simulink library "vhcl4turbAndrewMess_cl"  (R2022a)
settings: Solver=VariableStepAuto  StartTime=0.0  StopTime=10.0  RelTol=1e-3
undefined symbols (not defined in the file): env, thrSwitch, VEHICLE, vhcl, XiTotA, XiTotD
libraries: vrlib x4, addedMass_cl x1, pathFollowingCtrlAoATurbDiscrete_cl x1, dynamicPressure_ul x1, courseFollowLookAhead_cl x1, sharedutil x1, gnd2TanRotation_ul x1, pathGeometry_ul x1, velocityAngle_ul x1, alphaBeta_ul x1, dragTurbine x1, Copy_of_fluidDynamicSurface_cl x1
settings Model: Creator=mcobb  LastModifiedBy=adabney
settings SolverCC: AlgebraicLoopSolver=TrustRegion
settings DataIOCC: ReturnWorkspaceOutputs=off
settings DebuggingCC: UnconnectedInputMsg=warning  UnconnectedOutputMsg=warning  UnconnectedLineMsg=warning  SFMachineParentedDataDiag=warning  ArithmeticOperatorsInVariantConditions=warning
settings SFSimCC: CustomCodeUndefinedFunction=UseInterfaceOnly

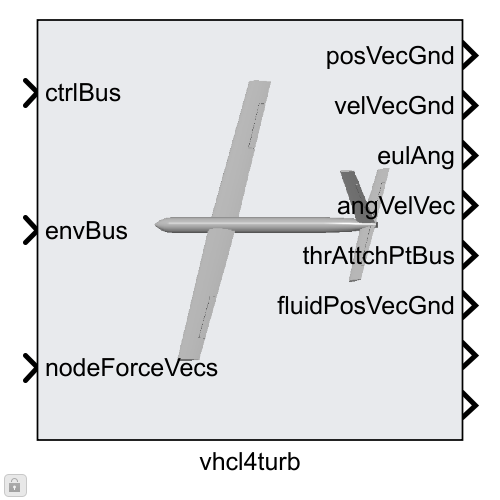
[thumbnail: Simulink's stored preview of the top-level diagram]
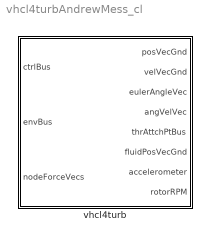
== system vhcl4turbAndrewMess_cl ==
  vhcl4turb : Subsystem  VariantControl=strcmpi(VEHICLE,'vehicleManta')  mask{vcl=vhcl, rho=env.water.density.Value, grav=env.gravAccel.Value}
      mask prompts: vcl "Vehicle"; rho "Density"; grav "Gravity"
      mask init:
      | numTurb = vcl.numTurbines.Value;
      | 
      | if numTurb == 0
      |     turbInd = [];
      |     gradInd = [6:11];
      | else
      |     turbInd = [1:numTurb]+5;
      |     gradInd = [6:11]+numTurb;
      | end
      | 
      | flowPoll = ones(1,numTurb+11);
      mask DialogControl Container9 Prompt: General
      mask DialogControl Container5 Prompt: Vehicle object (OCT.vehicle)
      mask DialogControl ParameterGroupVar Prompt: Environment Object (OCT.env)
      mask Display:
      | image('kite2.PNG',[0 0 700 700]/4,'on')
      | 
      | port_label('input',1,'ctrlBus')
      | port_label('input',2,'envBus')
      | port_label('input',3,'nodeForceVecs')
      | 
      | port_label('output',1,'posVecGnd')
      | port_label('output',2,'velVecGnd')
      | port_label('output',3,'eulAng')
      | port_label('output',4,'angVelVec')
      | port_label('output',5,'thrAttchPtBus')
      | port_label('output',6,'fluidPosVecGnd')

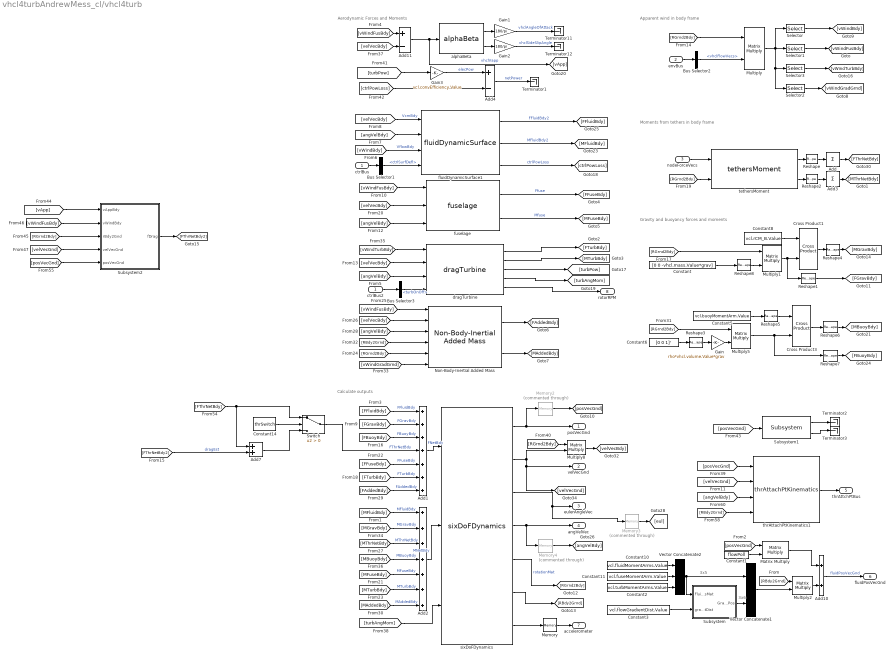
== system vhcl4turbAndrewMess_cl/vhcl4turb ==
  note: 3x6
  note: 3x5
  note: Calculate outputs
  note: Apparent wind in body frame
  note: Gravity and buoyancy forces and moments
  note: Moments from tethers in body frame
  note: Aerodynamic Forces and Moments
  ctrlBus : Inport  OutDataTypeStr=Bus: fltCtrlBus
  envBus : Inport  Port=2  OutDataTypeStr=Bus: envBus
  nodeForceVecs : Inport  Port=3
  Add : Sum  Inputs=+  CollapseMode=Specified dimension  CollapseDim=2
  Add1 : Sum  Inputs=+++++++
  Add10 : Sum
  Add11 : Sum  Inputs=+-
  Add2 : Sum  Inputs=+++++++
  Add3 : Sum  Inputs=+  CollapseMode=Specified dimension  CollapseDim=2
  Add4 : Sum  Inputs=+-
  Add7 : Sum
  Bus Selector1 : BusSelector  OutputSignals=ctrlSurfDefl
  Bus Selector2 : BusSelector  OutputSignals=vhclFlowVecs
  Bus Selector3 : BusSelector  OutputSignals=turbOnOff
  Constant : Constant  Value=[0 0 -vhcl.mass.Value*grav]
  Constant1 : Constant  Value=flowPoll  VectorParams1D=off
  Constant10 : Constant  Value=vcl.fluidMomentArms.Value
  Constant11 : Constant  Value=vcl.fuseMomentArm.Value
  Constant14 : Constant  Value=thrSwitch
  Constant2 : Constant  Value=vcl.turbMomentArms.Value
  Constant3 : Constant  Value=vcl.flowGradientDist.Value
  Constant5 : Constant  Value=vcl.buoyMomentArm.Value
  Constant6 : Constant  Value=[0 0 1]'
  Constant8 : Constant  Value=vcl.rCM_B.Value
  Cross Product1 : vrlib/Utilities/Cross Product
  Cross Product3 : vrlib/Utilities/Cross Product
  Gain : Gain  Gain=rho*vhcl.volume.Value*grav
  Gain1 : Gain  Gain=180/pi
  Gain2 : Gain  Gain=180/pi
  Gain3 : Gain  Gain=vcl.convEfficiency.Value
  Matrix Multiply : Product  Multiplication=Matrix(*)
  Memory : Memory
  Memory2 : Memory  Commented=through  InitialCondition=vcl.initPosVecGnd.Value
  Memory3 : Memory  Commented=through  InitialCondition=vcl.initEulAng.Value
  Memory4 : Memory  Commented=through  InitialCondition=vcl.initAngVelVec.Value
  Multiply{,1..2,5,8} (5 alike) : Product  Multiplication=Matrix(*)
  Non-Body-Inertial Added Mass : addedMass_cl/Non-Body-Inertial Added Mass  MaMat=vcl.Ma6x6_LE.Value  rB_LE=vcl.rB_LE.Value  gradDist=vcl.flowGradientDist.Value
  Reshape : Reshape  OutputDimensionality=Customize  OutputDimensions=[3 vcl.numTethers.Value]
  Reshape{1,3..8} (7 alike) : Reshape  OutputDimensionality=Column vector (2-D)
  Reshape2 : Reshape  OutputDimensionality=Customize  OutputDimensions=[3 vcl.numTethers.Value]
  Selector : Selector  NumberOfDimensions=2  InputPortWidth=3  IndexOptions=Select all,Index vector (dialog)  Indices=[1 3],1:4  OutputSizes=1,1
  Selector1 : Selector  NumberOfDimensions=2  InputPortWidth=3  IndexOptions=Select all,Index vector (dialog)  Indices=[1 3],5  OutputSizes=1,1
  Selector2 : Selector  NumberOfDimensions=2  InputPortWidth=3  IndexOptions=Select all,Index vector (dialog)  Indices=[1 3],gradInd  OutputSizes=1,1
  Selector3 : Selector  NumberOfDimensions=2  InputPortWidth=3  IndexOptions=Select all,Index vector (dialog)  Indices=[1 3],turbInd  OutputSizes=1,1
  Subsystem : Subsystem
  Subsystem1 : pathFollowingCtrlAoATurbDiscrete_cl/pathFollowingCtrlAoATurbDiscrete/Subsystem  SystemSampleTime=-1  VariantActivationTime=update diagram  Latency=0  AutoFrameSizeCalculation=off
  Subsystem2 : Subsystem  mask{vcl=vcl}
      mask prompts: vcl "Vehicle"
  Switch : Switch  Criteria=u2 > Threshold  SaturateOnIntegerOverflow=off  InputSameDT=off
  Terminator{1..3,11..12} (5 alike) : Terminator
  Vector Concatenate1 : Concatenate  Mode=Multidimensional array  ConcatenateDimension=2
  Vector Concatenate2 : Concatenate  NumInputs=3  Mode=Multidimensional array  ConcatenateDimension=2
  alphaBeta : alphaBeta_ul/alphaBeta  SystemSampleTime=-1  VariantActivationTime=update diagram  Latency=0  AutoFrameSizeCalculation=off
  ctrlBus2 : InportShadow  OutDataTypeStr=Bus: fltCtrlBus
  dragTurbine : dragTurbine/dragTurbine  vhcl=vcl  thr=0
  fluidDynamicSurface1 : Copy_of_fluidDynamicSurface_cl/fluidDynamicSurface  vcl=vcl  fluidDensity=env.water.density.Value  fluidMomentArms=vcl.fluidMomentArms.Value  fluidRefArea=vcl.fluidRefArea.Value  wingTips=vcl.wingTipPositions.Value
  fuselage : fuselage_cl/fuselage  momArm=vcl.fuseMomentArm.Value  fus=vcl.fuse  fusRhoDa=rho
  sixDoFDynamics : sixDoFDynamics_cl/sixDoFDynamics  vcl=vcl
  tethersMoment : tethersMoment_cl/tethersMoment  arms=vcl.struct('OCT.thrAttch')
  thrAttachPtKinematics1 : thrAttachPtKinematics_ul/thrAttachPtKinematics  atchPts=vcl.struct('OCT.thrAttch')
  posVecGnd : Outport  VectorParamsAs1DForOutWhenUnconnected=off
  velVecGnd : Outport  Port=2  VectorParamsAs1DForOutWhenUnconnected=off
  eulerAngleVec : Outport  Port=3  VectorParamsAs1DForOutWhenUnconnected=off
  angVelVec : Outport  Port=4  VectorParamsAs1DForOutWhenUnconnected=off
  thrAttchPtBus : Outport  Port=5  VectorParamsAs1DForOutWhenUnconnected=off
  fluidPosVecGnd : Outport  Port=6  VectorParamsAs1DForOutWhenUnconnected=off
  accelerometer : Outport  Port=7
  rotorRPM : Outport  Port=8
  wires:
  sixDoFDynamics/3 -> Memory3/1, eulerAngleVec/1
  sixDoFDynamics/1 -> Memory2/1, posVecGnd/1
  sixDoFDynamics/2 -> [velVecGnd], velVecGnd/1, Multiply8/2
  thrAttachPtKinematics1/1 -> thrAttchPtBus/1
  [vWindFusBdy] -> fuselage/1
  [velVecBdy] -> fuselage/2
  [angVelBdy] -> fuselage/3
  [vWindTurbBdy] -> dragTurbine/1
  [velVecBdy] -> dragTurbine/2
  [angVelBdy] -> dragTurbine/3
  [vWindFusBdy] -> Non-Body-Inertial Added Mass/1
  [velVecBdy] -> Non-Body-Inertial Added Mass/2
  [angVelBdy] -> Non-Body-Inertial Added Mass/3
  [RBdy2Grnd] -> Non-Body-Inertial Added Mass/4
  [RGrnd2Bdy] -> Non-Body-Inertial Added Mass/5
  [vWindGradGrnd] -> Non-Body-Inertial Added Mass/6
  Constant6/1 -> Reshape3/1
  Reshape3/1 -> Gain/1
  [RGrnd2Bdy] -> Multiply5/1
  Gain/1 -> Multiply5/2
  Constant5/1 -> Reshape5/1
  Reshape5/1 -> Cross Product3/1
  Cross Product3/1 -> Reshape6/1
  Reshape6/1 -> [MBuoyBdy]
  Multiply5/1 -> Reshape7/1, Cross Product3/2
  Reshape7/1 -> [FBuoyBdy]
  Reshape1/1 -> [FGravBdy]
  Multiply1/1 -> Reshape1/1, Cross Product1/2
  fuselage/1 -> [FFuseBdy]  "Ffuse"
  fuselage/2 -> [MFuseBdy]  "Mfuse"
  Constant/1 -> Reshape8/1
  [RGrnd2Bdy] -> Multiply1/1
  Reshape8/1 -> Multiply1/2
  Constant8/1 -> Cross Product1/1
  Cross Product1/1 -> Reshape4/1
  Reshape4/1 -> [MGravBdy]
  [RGrnd2Bdy] -> tethersMoment/2
  nodeForceVecs/1 -> tethersMoment/1
  tethersMoment/1 -> Reshape/1
  tethersMoment/2 -> Reshape2/1
  Reshape/1 -> Add/1
  Reshape2/1 -> Add3/1
  Add/1 -> [FThrNetBdy]
  Add3/1 -> [MThrNetBdy]
  [RGrnd2Bdy] -> Multiply/1
  envBus/1 -> Bus Selector2/1
  Bus Selector2/1 -> Multiply/2  "<vhclFlowVecs>"
  Multiply/1 -> Selector/1, Selector2/1, Selector3/1, Selector1/1
  Selector/1 -> [vWindBdy]
  Selector1/1 -> [vWindFusBdy]
  Selector2/1 -> [vWindGradGrnd]
  [RGrnd2Bdy] -> Multiply8/1
  Multiply8/1 -> [velVecBdy]
  [FFluidBdy] -> Add1/1  "FFluidBdy"
  [FGravBdy] -> Add1/2  "FGravBdy"
  [FBuoyBdy] -> Add1/3  "FBuoyBdy"
  Switch/1 -> Add1/4  "FThrNetBdy"
  [FFuseBdy] -> Add1/5  "FFuseBdy"
  [FTurbBdy] -> Add1/6  "FTurbBdy"
  [FAddedBdy] -> Add1/7  "FAddedBdy"
  Add1/1 -> sixDoFDynamics/1  "FNetBdy"
  [MFluidBdy] -> Add2/1  "MFluidBdy"
  [MGravBdy] -> Add2/2  "MGravBdy"
  [MThrNetBdy] -> Add2/3  "MThrNetBdy"
  [MBuoyBdy] -> Add2/4  "MBuoyBdy"
  [MFuseBdy] -> Add2/5  "MFuseBdy"
  [MTurbBdy] -> Add2/6  "MTurbBdy"
  [MAddedBdy] -> Add2/7  "MAddedBdy"
  Add2/1 -> sixDoFDynamics/2  "MNetBdy"
  sixDoFDynamics/5 -> [RGrnd2Bdy]  "rotationMat"
  sixDoFDynamics/6 -> [RBdy2Grnd]
  [posVecGnd] -> thrAttachPtKinematics1/1
  [velVecGnd] -> thrAttachPtKinematics1/2
  [angVelBdy] -> thrAttachPtKinematics1/3
  [RBdy2Grnd] -> thrAttachPtKinematics1/4
  Constant10/1 -> Vector Concatenate2/1
  Constant11/1 -> Vector Concatenate2/2
  Vector Concatenate2/1 -> Vector Concatenate1/1, Subsystem/1(FluidCentPosMat)
  Constant3/1 -> Subsystem/2(gradientDist)
  Subsystem/1(GradientFlowPos) -> Vector Concatenate1/2
  sixDoFDynamics/4 -> Memory4/1, angVelVec/1
  Vector Concatenate1/1 -> Multiply2/2
  [RBdy2Grnd] -> Multiply2/1
  Multiply2/1 -> Add10/2
  Matrix Multiply/1 -> Add10/1
  Add10/1 -> fluidPosVecGnd/1  "fluidPosVecGnd"
  Constant1/1 -> Matrix Multiply/2
  [posVecGnd] -> Matrix Multiply/1
  Bus Selector3/1 -> dragTurbine/4  "<turbOnOff>"
  ctrlBus2/1 -> Bus Selector3/1
  Constant2/1 -> Vector Concatenate2/3
  Selector3/1 -> [vWindTurbBdy]
  dragTurbine/1 -> [FTurbBdy]
  dragTurbine/2 -> [MTurbBdy]
  dragTurbine/3 -> [turbPow]
  dragTurbine/4 -> [turbAngMom]
  dragTurbine/5 -> rotorRPM/1
  fluidDynamicSurface1/1 -> [FFluidBdy]  "FFluidBdy2"
  Gain3/1 -> Add4/1  "elecPow"
  [ctrlPowLoss] -> Add4/2
  [turbPow] -> Gain3/1
  fluidDynamicSurface1/3 -> [ctrlPowLoss]  "ctrlPowLoss"
  [angVelBdy] -> fluidDynamicSurface1/2
  [vWindBdy] -> fluidDynamicSurface1/3  "VflowBdy"
  [velVecBdy] -> fluidDynamicSurface1/1  "VcmBdy"
  fluidDynamicSurface1/2 -> [MFluidBdy]  "MFluidBdy2"
  Bus Selector1/1 -> fluidDynamicSurface1/4  "<ctrlSurfDefl>"
  Gain2/1 -> Terminator12/1  "vhclSideSlipAngle"
  alphaBeta/1 -> Gain1/1
  Add4/1 -> Terminator1/1  "netPower"
  Gain1/1 -> Terminator11/1  "vhclAngleOfAttack"
  [vWindFusBdy] -> Add11/1
  Add11/1 -> [vApp], alphaBeta/1  "vhclVapp"
  alphaBeta/2 -> Gain2/1
  ctrlBus/1 -> Bus Selector1/1
  Memory/1 -> accelerometer/1
  sixDoFDynamics/7 -> Memory/1
  [turbAngMom] -> sixDoFDynamics/3
  [posVecGnd] -> Subsystem1/1
  Subsystem1/1 -> Terminator2/1
  Subsystem1/2 -> Terminator3/1
  Non-Body-Inertial Added Mass/1 -> [FAddedBdy]
  Non-Body-Inertial Added Mass/2 -> [MAddedBdy]
  [velVecBdy] -> Add11/2
  Memory2/1 -> [posVecGnd]
  Memory3/1 -> [eul]
  Memory4/1 -> [angVelBdy]
  [FThrNetBdy2] -> Add7/2  "dragEst"
  Constant14/1 -> Switch/2
  [FThrNetBdy] -> Add7/1, Switch/1
  Add7/1 -> Switch/3
  [vApp] -> Subsystem2/1(vAppBdy)
  [vWindFusBdy] -> Subsystem2/2(vWindBdy)
  [velVecGnd] -> Subsystem2/4(velVecGnd)
  [posVecGnd] -> Subsystem2/5(posVecGnd)
  [RGrnd2Bdy] -> Subsystem2/3(rBdy2Gnd)
  Subsystem2/1(fDrag) -> [FThrNetBdy2]

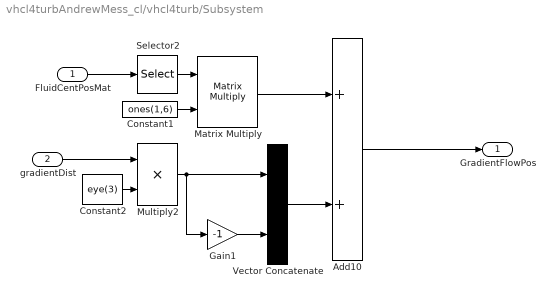
== system vhcl4turbAndrewMess_cl/vhcl4turb/Subsystem ==
  FluidCentPosMat : Inport
  gradientDist : Inport  Port=2
  Add10 : Sum
  Constant1 : Constant  Value=ones(1,6)  VectorParams1D=off
  Constant2 : Constant  Value=eye(3)
  Gain1 : Gain  Gain=-1
  Matrix Multiply : Product  Multiplication=Matrix(*)
  Multiply2 : Product
  Selector2 : Selector  NumberOfDimensions=2  InputPortWidth=3  IndexOptions=Select all,Index vector (dialog)  Indices=[1 3],5  OutputSizes=1,1
  Vector Concatenate : Concatenate  Mode=Multidimensional array  ConcatenateDimension=2
  GradientFlowPos : Outport  VectorParamsAs1DForOutWhenUnconnected=off
  wires:
  FluidCentPosMat/1 -> Selector2/1
  Vector Concatenate/1 -> Add10/2
  Selector2/1 -> Matrix Multiply/1
  Multiply2/1 -> Gain1/1, Vector Concatenate/1
  Constant1/1 -> Matrix Multiply/2
  Matrix Multiply/1 -> Add10/1
  Gain1/1 -> Vector Concatenate/2
  Constant2/1 -> Multiply2/2
  Add10/1 -> GradientFlowPos/1
  gradientDist/1 -> Multiply2/1

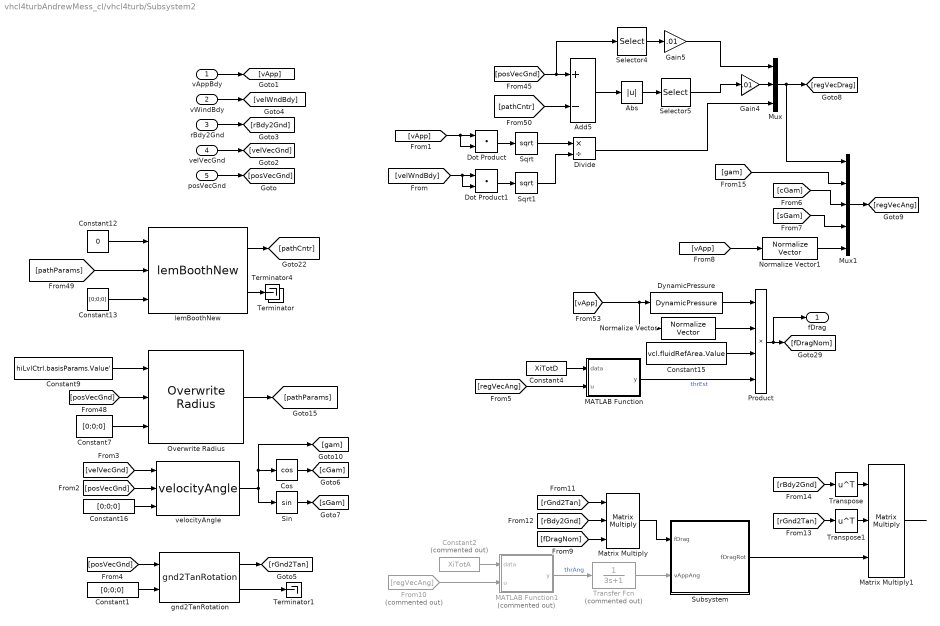
== system vhcl4turbAndrewMess_cl/vhcl4turb/Subsystem2 ==
  vAppBdy : Inport
  vWindBdy : Inport  Port=2
  rBdy2Gnd : Inport  Port=3
  velVecGnd : Inport  Port=4
  posVecGnd : Inport  Port=5
  Abs : Abs  SaturateOnIntegerOverflow=off
  Add5 : Sum  Inputs=+-
  Constant{1,7,13,16} (4 alike) : Constant  Value=[0;0;0]  VectorParams1D=off
  Constant12 : Constant  Value=0
  Constant15 : Constant  Value=vcl.fluidRefArea.Value
  Constant2 : Constant  Commented=on  Value=XiTotA
  Constant4 : Constant  Value=XiTotD
  Constant9 : Constant  Value=hiLvlCtrl.basisParams.Value'  VectorParams1D=off
  Cos : Trigonometry  Operator=cos
  Divide : Product  Inputs=*/
  Dot Product : DotProduct  OutDataTypeStr=Inherit: Inherit via internal rule
  Dot Product1 : DotProduct  OutDataTypeStr=Inherit: Inherit via internal rule
  DynamicPressure : dynamicPressure_ul/DynamicPressure  rho=1000
  From10 : From  Commented=on  GotoTag=regVecAng
  Gain4 : Gain  Gain=.01
  Gain5 : Gain  Gain=.01
  MATLAB Function : MATLAB Function  TreatAsAtomicUnit=on
  MATLAB Function1 : MATLAB Function  Commented=on  TreatAsAtomicUnit=on
  Matrix Multiply : Product  Inputs=3  Multiplication=Matrix(*)
  Matrix Multiply1 : Product  Inputs=3  Multiplication=Matrix(*)
  Mux : Mux  Inputs=3
  Mux1 : Mux  Inputs=5
  Normalize Vector : vrlib/Utilities/Normalize Vector  maxzero=0
  Normalize Vector1 : vrlib/Utilities/Normalize Vector  maxzero=0
  Overwrite Radius : courseFollowLookAhead_cl/courseFollowLookAhead/Overwrite Radius  SystemSampleTime=-1  VariantActivationTime=update diagram  Latency=0  AutoFrameSizeCalculation=off
  Product : Product  Inputs=4
  Selector4 : Selector  InputPortWidth=3  IndexOptions=Index vector (dialog)  Indices=3  OutputSizes=1
  Selector5 : Selector  InputPortWidth=3  IndexOptions=Index vector (dialog)  Indices=[2 3]  OutputSizes=1
  Sin : Trigonometry
  Sqrt : Sqrt
  Sqrt1 : Sqrt
  Subsystem : Subsystem
  Terminator : Terminator
  Terminator1 : Terminator
  Terminator4 : Terminator
  Transfer Fcn : TransferFcn  Commented=on  Denominator=[3 1]
  Transpose : Math  Operator=transpose
  Transpose1 : Math  Operator=transpose
  gnd2TanRotation : gnd2TanRotation_ul/gnd2TanRotation  SystemSampleTime=-1  VariantActivationTime=update diagram  Latency=0  AutoFrameSizeCalculation=off
  lemBoothNew : pathGeometry_ul/pathGeometry/lemBoothNew  SystemSampleTime=-1  VariantControl=VSS_pathGeometry_lemBoothNew  VariantActivationTime=update diagram  Latency=0  AutoFrameSizeCalculation=off
  velocityAngle : velocityAngle_ul/velocityAngle  SystemSampleTime=-1  VariantActivationTime=update diagram  Latency=0  AutoFrameSizeCalculation=off
  fDrag : Outport
  wires:
  [posVecGnd] -> Overwrite Radius/2
  lemBoothNew/2 -> Terminator4/1
  Overwrite Radius/1 -> [pathParams]
  Selector4/1 -> Gain5/1
  Abs/1 -> Selector5/1
  Constant12/1 -> lemBoothNew/1
  Gain4/1 -> Mux/2
  Constant13/1 -> lemBoothNew/3
  Add5/1 -> Abs/1
  Dot Product1/1 -> Sqrt1/1
  lemBoothNew/1 -> [pathCntr]
  Gain5/1 -> Mux/1
  Sqrt1/1 -> Divide/2
  Sqrt/1 -> Divide/1
  Dot Product/1 -> Sqrt/1
  velocityAngle/1 -> [gam], Cos/1, Sin/1
  Divide/1 -> Mux/3
  [posVecGnd] -> Selector4/1, Add5/1
  Constant16/1 -> velocityAngle/3
  Constant7/1 -> Overwrite Radius/3
  Constant9/1 -> Overwrite Radius/1
  Mux/1 -> Mux1/1, [regVecDrag]
  [pathCntr] -> Add5/2
  [pathParams] -> lemBoothNew/2
  Selector5/1 -> Gain4/1
  posVecGnd/1 -> [posVecGnd]
  vAppBdy/1 -> [vApp]
  vWindBdy/1 -> [velWndBdy]
  [velWndBdy] -> Dot Product1/2, Dot Product1/1
  [vApp] -> Dot Product/2, Dot Product/1
  rBdy2Gnd/1 -> [rBdy2Gnd]
  velVecGnd/1 -> [velVecGnd]
  [posVecGnd] -> velocityAngle/2
  [velVecGnd] -> velocityAngle/1
  Cos/1 -> [cGam]
  Sin/1 -> [sGam]
  gnd2TanRotation/1 -> [rGnd2Tan]
  [posVecGnd] -> gnd2TanRotation/1
  Constant1/1 -> gnd2TanRotation/2
  gnd2TanRotation/2 -> Terminator1/1
  [vApp] -> Normalize Vector/1, DynamicPressure/1
  Product/1 -> fDrag/1, [fDragNom]
  Normalize Vector/1 -> Product/2
  Constant15/1 -> Product/3
  MATLAB Function/1(y) -> Product/4  "thrEst"
  DynamicPressure/1 -> Product/1
  Constant4/1 -> MATLAB Function/1(data)
  [regVecAng] -> MATLAB Function/2(u)
  [cGam] -> Mux1/3
  [sGam] -> Mux1/4
  [vApp] -> Normalize Vector1/1
  Mux1/1 -> [regVecAng]
  From10/1 -> MATLAB Function1/2(u)
  Constant2/1 -> MATLAB Function1/1(data)
  MATLAB Function1/1(y) -> Transfer Fcn/1  "thrAng"
  Subsystem/1(fDragRot) -> Matrix Multiply1/3
  [fDragNom] -> Matrix Multiply/3
  [rBdy2Gnd] -> Matrix Multiply/2
  [rGnd2Tan] -> Matrix Multiply/1
  Matrix Multiply/1 -> Subsystem/1(fDrag)
  [rBdy2Gnd] -> Transpose/1
  Transpose/1 -> Matrix Multiply1/1
  [rGnd2Tan] -> Transpose1/1
  Transpose1/1 -> Matrix Multiply1/2
  Matrix Multiply1/1 -> ?
  [gam] -> Mux1/2
  Normalize Vector1/1 -> Mux1/5
  Transfer Fcn/1 -> Subsystem/2(vAppAng)

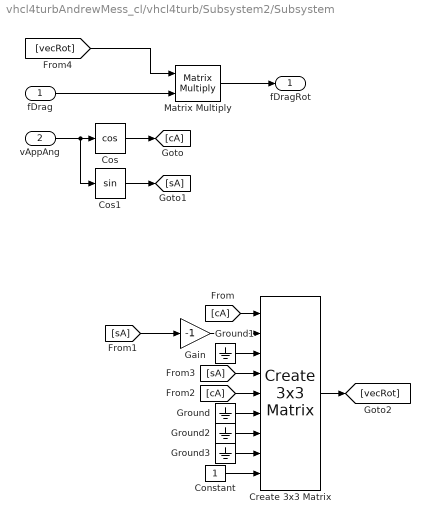
== system vhcl4turbAndrewMess_cl/vhcl4turb/Subsystem2/Subsystem ==
  fDrag : Inport
  vAppAng : Inport  Port=2
  Constant : Constant
  Cos : Trigonometry  Operator=cos
  Cos1 : Trigonometry
  Create 3x3 Matrix : sharedutil/Create 3x3 Matrix  aMode=aMode
      settings: SourceProductBaseCode=AE,PW,DR,MT,VE
  Gain : Gain  Gain=-1
  Ground{,1..3} (4 alike) : Ground
  Matrix Multiply : Product  Multiplication=Matrix(*)
  fDragRot : Outport
  wires:
  fDrag/1 -> Matrix Multiply/2
  vAppAng/1 -> Cos1/1, Cos/1
  Cos/1 -> [cA]
  Cos1/1 -> [sA]
  Constant/1 -> Create 3x3 Matrix/9
  Ground/1 -> Create 3x3 Matrix/6
  Ground1/1 -> Create 3x3 Matrix/3
  [cA] -> Create 3x3 Matrix/1
  [sA] -> Gain/1
  [cA] -> Create 3x3 Matrix/5
  [sA] -> Create 3x3 Matrix/4
  Ground3/1 -> Create 3x3 Matrix/8
  Ground2/1 -> Create 3x3 Matrix/7
  Create 3x3 Matrix/1 -> [vecRot]
  [vecRot] -> Matrix Multiply/1
  Matrix Multiply/1 -> fDragRot/1
  Gain/1 -> Create 3x3 Matrix/2

== matlab function vhcl4turbAndrewMess_cl/vhcl4turb/Subsystem2/MATLAB Function1 ==
  data: data input; u input; y output size=[1,1]
function y   = fcn(data, u)
%Estimate Tether Drag using output of a sequential least squares fit for a
%non-linear regressor vector

%Build Regressor Vector
nVars = numel(u);
ind = 1;
n = size(data);
yout = zeros(1,n(1));

for i=1:nVars
    yout(ind) = u(i);
    ind = ind+1;
end

% poly order 2
for i=1:nVars
    for j=i:nVars
        yout(ind) = u(i).*u(j);
        ind = ind+1;
    end
end


y = yout*data;
% y = min([y 1]);
% y = max([y 0]);

== matlab function vhcl4turbAndrewMess_cl/vhcl4turb/Subsystem2/MATLAB Function ==
  data: data input; u input; y output size=[1,1]
function y   = fcn(data, u)
%Estimate Tether Drag using output of a sequential least squares fit for a
%non-linear regressor vector

%Build Regressor Vector
nVars = numel(u);
ind = 1;
n = size(data);
yout = zeros(1,n(1));

for i=1:nVars
    yout(ind) = u(i);
    ind = ind+1;
end

% poly order 2
for i=1:nVars
    for j=i:nVars
        yout(ind) = u(i).*u(j);
        ind = ind+1;
    end
end



y = yout*data;
y = min([y 1]);
y = max([y 0]);
